simulink model "gm_Custom_DA_FIR3"  (R2023b)
settings: Solver=FixedStepDiscrete  StartTime=0.0  StopTime=10.0  RelTol=1e-3
libraries: hdlsllib x40
settings Model: Creator=adity_6z2h70p  LastModifiedBy=adity_6z2h70p
settings OptimizationCC: BlockReduction=off  ConditionallyExecuteInputs=off  DefaultParameterBehavior=Inlined  InheritOutputTypeSmallerThanSingle=on
settings DebuggingCC: AlgebraicLoopMsg=error  InheritedTsInSrcMsg=none  SingleTaskRateTransMsg=error
settings HardwareCC: ProdBitPerPointer=32  ProdBitPerSizeT=32  ProdBitPerPtrDiffT=32  ProdLargestAtomicFloat=None  ProdIntDivRoundTo=Undefined  ProdEndianess=Unspecified  ProdWordSize=32  ProdHWDeviceType=ASIC/FPGA->ASIC/FPGA  TargetBitPerPointer=64  TargetBitPerSizeT=64  TargetBitPerPtrDiffT=64  TargetLongLongMode=on  TargetIntDivRoundTo=Zero  TargetEndianess=LittleEndian  TargetWordSize=64  TargetHWDeviceType=Custom Processor->MATLAB Host Computer  ProdEqTarget=off

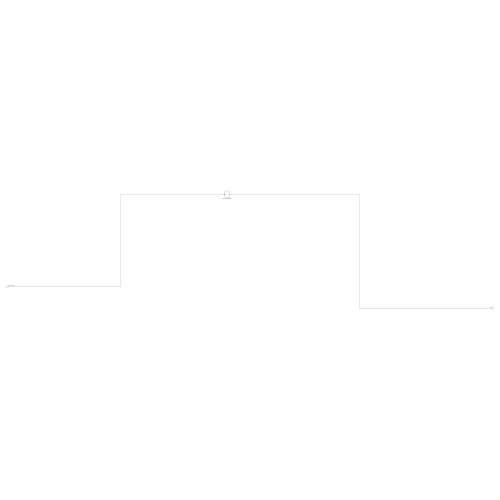
[thumbnail: Simulink's stored preview of the top-level diagram]
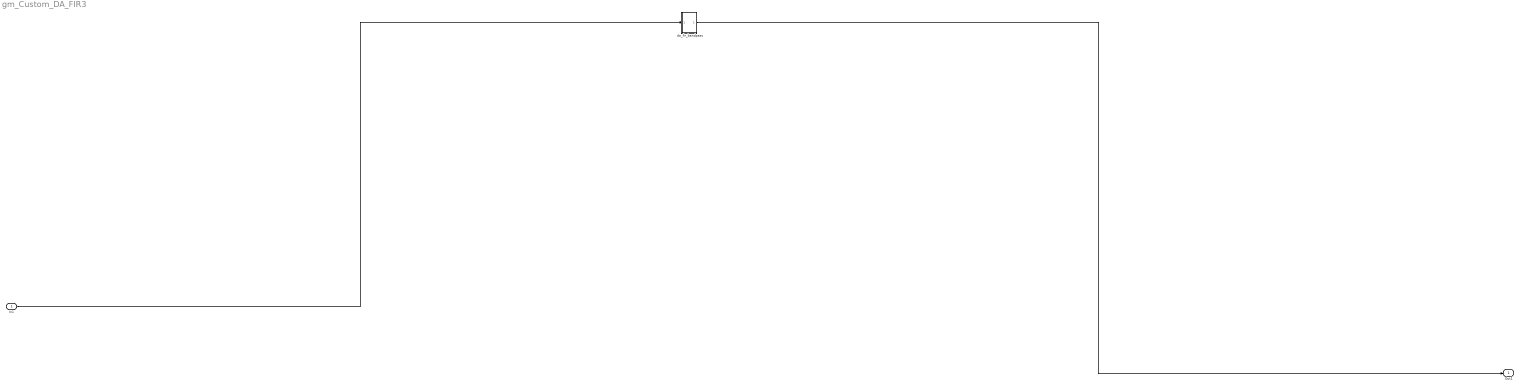
== system gm_Custom_DA_FIR3 ==
  In1 : Inport  OutDataTypeStr=fixdt(1,16,15)
  da_fir_bandpass : Subsystem
  Out1 : Outport
  wires:
  da_fir_bandpass/1(Out1) -> Out1/1
  In1/1 -> da_fir_bandpass/1(In1)

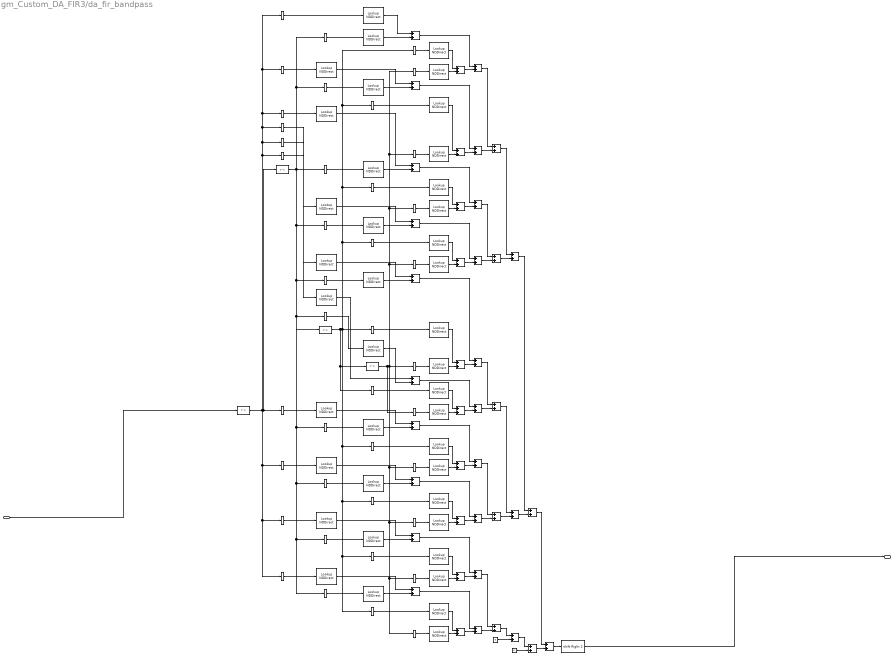
== system gm_Custom_DA_FIR3/da_fir_bandpass ==
  In1 : Inport
  Adder_S1_{1..20} (20 alike) : Sum
  Adder_S2_{1..10} (10 alike) : Sum
  Adder_S3_{1..5} (5 alike) : Sum
  Adder_S4_1 : Sum
  Adder_S4_2 : Sum
  Adder_S4_3 : Sum
  Adder_S5_1 : Sum
  Adder_S5_2 : Sum
  Adder_S6_1 : Sum
  BitSlice_Chunk_{1..40} (40 alike) : hdlsllib/Logic and Bit Operations/Bit Slice  lidx=3  ridx=0
  ConstZero_S4_3 : Constant  Value=0  OutDataTypeStr=fixdt(1,16,15)  SampleTime=-1
  ConstZero_S5_2 : Constant  Value=0  OutDataTypeStr=fixdt(1,16,15)  SampleTime=-1
  Delay_{1..4} (4 alike) : Delay  DelayLength=1
  LUT_Chunk_{1,5,8..9,11,14,18,22,26,32,35..36,39} (13 alike) : LookupNDDirect  NumberOfTableDimensions=1  Table=[0 -1 -1 -1 -1 -1 -1 -1 -1 -1 -1 -1 -1 -1 -1 -1]  TableDataTypeStr=fixdt(1,16,15)
  LUT_Chunk_10 : LookupNDDirect  NumberOfTableDimensions=1  Table=[0 0.999969482421875 0.999969482421875 0.999969482421875 0.999969482421875 0.999969482421875 0.999969482421875 0.999969482421875 -1 -1 0.999969482421875 0.999969482421875 0.999969482421875 0.999969482421875 0.999969482421875 0.999969482421875]  TableDataTypeStr=fixdt(1,16,15)
  LUT_Chunk_{3,7,12..13,16,20,24,28,34,37..38} (11 alike) : LookupNDDirect  NumberOfTableDimensions=1  Table=[0 0.999969482421875 0.999969482421875 0.999969482421875 0.999969482421875 0.999969482421875 0.999969482421875 0.999969482421875 0.999969482421875 0.999969482421875 0.999969482421875 0.999969482421875 0.999969482421875 0.999969482421875 0.999969482421875 0.999969482421875]  TableDataTypeStr=fixdt(1,16,15)
  LUT_Chunk_15 : LookupNDDirect  NumberOfTableDimensions=1  Table=[0 -1 -1 -1 -1 -1 -1 -1 0.999969482421875 -1 -1 -1 -1 -1 -1 -1]  TableDataTypeStr=fixdt(1,16,15)
  LUT_Chunk_17 : LookupNDDirect  NumberOfTableDimensions=1  Table=[0 0.999969482421875 0.999969482421875 0.999969482421875 0.999969482421875 0.999969482421875 0.999969482421875 0.999969482421875 -1 0.999969482421875 0.999969482421875 0.999969482421875 -1 0.999969482421875 0.999969482421875 0.999969482421875]  TableDataTypeStr=fixdt(1,16,15)
  LUT_Chunk_19 : LookupNDDirect  NumberOfTableDimensions=1  Table=[0 -1 -1 -1 -1 -1 -1 -1 0.999969482421875 -1 -1 -1 0.999969482421875 -1 -1 -1]  TableDataTypeStr=fixdt(1,16,15)
  LUT_Chunk_2 : LookupNDDirect  NumberOfTableDimensions=1  Table=[0 -1 0.999969482421875 -1 0.999969482421875 0.999969482421875 0.999969482421875 0.999969482421875 0.999969482421875 0.999969482421875 0.999969482421875 0.999969482421875 0.999969482421875 0.999969482421875 0.999969482421875 0.999969482421875]  TableDataTypeStr=fixdt(1,16,15)
  LUT_Chunk_21 : LookupNDDirect  NumberOfTableDimensions=1  Table=[0 0.999969482421875 0.999969482421875 0.999969482421875 -1 0.999969482421875 0.999969482421875 0.999969482421875 -1 0.999969482421875 -1 0.999969482421875 -1 0.999969482421875 -1 0.999969482421875]  TableDataTypeStr=fixdt(1,16,15)
  LUT_Chunk_23 : LookupNDDirect  NumberOfTableDimensions=1  Table=[0 -1 -1 -1 0.999969482421875 -1 -1 -1 0.999969482421875 -1 0.999969482421875 -1 0.999969482421875 0.999969482421875 0.999969482421875 -1]  TableDataTypeStr=fixdt(1,16,15)
  LUT_Chunk_25 : LookupNDDirect  NumberOfTableDimensions=1  Table=[0 0.999969482421875 0.999969482421875 0.999969482421875 -1 0.999969482421875 -1 0.999969482421875 -1 -1 -1 0.999969482421875 -1 -1 -1 -1]  TableDataTypeStr=fixdt(1,16,15)
  LUT_Chunk_27 : LookupNDDirect  NumberOfTableDimensions=1  Table=[0 -1 0.999969482421875 -1 0.999969482421875 -1 0.999969482421875 -1 0.999969482421875 0.999969482421875 0.999969482421875 0.999969482421875 0.999969482421875 0.999969482421875 0.999969482421875 0.999969482421875]  TableDataTypeStr=fixdt(1,16,15)
  LUT_Chunk_29 : LookupNDDirect  NumberOfTableDimensions=1  Table=[0 0.999969482421875 -1 0.999969482421875 -1 -1 -1 -1 -1 -1 -1 -1 -1 -1 -1 -1]  TableDataTypeStr=fixdt(1,16,15)
  LUT_Chunk_30 : LookupNDDirect  NumberOfTableDimensions=1  Table=[0 -1 -1 -1 0.999969482421875 -1 0.999969482421875 -1 0.999969482421875 -1 0.999969482421875 -1 0.999969482421875 -1 0.999969482421875 -1]  TableDataTypeStr=fixdt(1,16,15)
  LUT_Chunk_31 : LookupNDDirect  NumberOfTableDimensions=1  Table=[0 0.999969482421875 -1 -1 -1 -1 -1 -1 -1 -1 -1 -1 -1 -1 -1 -1]  TableDataTypeStr=fixdt(1,16,15)
  LUT_Chunk_33 : LookupNDDirect  NumberOfTableDimensions=1  Table=[0 -1 0.999969482421875 0.999969482421875 0.999969482421875 0.999969482421875 0.999969482421875 0.999969482421875 0.999969482421875 0.999969482421875 0.999969482421875 0.999969482421875 0.999969482421875 0.999969482421875 0.999969482421875 0.999969482421875]  TableDataTypeStr=fixdt(1,16,15)
  LUT_Chunk_4 : LookupNDDirect  NumberOfTableDimensions=1  Table=[0 0.999969482421875 -1 0.999969482421875 -1 -1 -1 -1 -1 -1 -1 -1 -1 -1 -1 -1]  TableDataTypeStr=fixdt(1,16,15)
  LUT_Chunk_40 : LookupNDDirect  NumberOfTableDimensions=1  Table=[0 -1 0 -1 0 -1 0 -1 0 -1 0 -1 0 -1 0 -1]  TableDataTypeStr=fixdt(1,16,15)
  LUT_Chunk_6 : LookupNDDirect  NumberOfTableDimensions=1  Table=[0 -1 0.999969482421875 0.999969482421875 0.999969482421875 0.999969482421875 0.999969482421875 0.999969482421875 0.999969482421875 0.999969482421875 0.999969482421875 0.999969482421875 0.999969482421875 0.999969482421875 0.999969482421875 0.999969482421875]  TableDataTypeStr=fixdt(1,16,15)
  Shift_Arithmetic_Scale : ArithShift  BitShiftNumber=2  BitShiftDirection=Right
  Out1 : Outport
  wires:
  LUT_Chunk_16/1 -> Adder_S1_8/2
  LUT_Chunk_31/1 -> Adder_S1_16/1
  Adder_S1_5/1 -> Adder_S2_3/1
  LUT_Chunk_37/1 -> Adder_S1_19/1
  BitSlice_Chunk_19/1 -> LUT_Chunk_19/1
  ConstZero_S5_2/1 -> Adder_S5_2/2
  Adder_S4_2/1 -> Adder_S5_1/2
  Adder_S2_7/1 -> Adder_S3_4/1
  LUT_Chunk_7/1 -> Adder_S1_4/1
  Adder_S1_17/1 -> Adder_S2_9/1
  Adder_S6_1/1 -> Shift_Arithmetic_Scale/1
  LUT_Chunk_8/1 -> Adder_S1_4/2
  Adder_S1_20/1 -> Adder_S2_10/2
  BitSlice_Chunk_30/1 -> LUT_Chunk_30/1
  BitSlice_Chunk_24/1 -> LUT_Chunk_24/1
  LUT_Chunk_20/1 -> Adder_S1_10/2
  LUT_Chunk_32/1 -> Adder_S1_16/2
  LUT_Chunk_21/1 -> Adder_S1_11/1
  LUT_Chunk_22/1 -> Adder_S1_11/2
  Adder_S1_10/1 -> Adder_S2_5/2
  Adder_S1_8/1 -> Adder_S2_4/2
  Adder_S1_18/1 -> Adder_S2_9/2
  Adder_S1_19/1 -> Adder_S2_10/1
  Adder_S2_10/1 -> Adder_S3_5/2
  BitSlice_Chunk_1/1 -> LUT_Chunk_1/1
  LUT_Chunk_40/1 -> Adder_S1_20/2
  LUT_Chunk_38/1 -> Adder_S1_19/2
  Adder_S3_2/1 -> Adder_S4_1/2
  LUT_Chunk_17/1 -> Adder_S1_9/1
  Adder_S1_16/1 -> Adder_S2_8/2
  LUT_Chunk_24/1 -> Adder_S1_12/2
  Adder_S3_3/1 -> Adder_S4_2/1
  Adder_S3_5/1 -> Adder_S4_3/1
  ConstZero_S4_3/1 -> Adder_S4_3/2
  LUT_Chunk_27/1 -> Adder_S1_14/1
  Adder_S2_8/1 -> Adder_S3_4/2
  LUT_Chunk_6/1 -> Adder_S1_3/2
  Adder_S5_1/1 -> Adder_S6_1/1
  Adder_S1_2/1 -> Adder_S2_1/2
  LUT_Chunk_35/1 -> Adder_S1_18/1
  LUT_Chunk_29/1 -> Adder_S1_15/1
  BitSlice_Chunk_5/1 -> LUT_Chunk_5/1
  Adder_S1_7/1 -> Adder_S2_4/1
  Adder_S1_3/1 -> Adder_S2_2/1
  LUT_Chunk_9/1 -> Adder_S1_5/1
  BitSlice_Chunk_23/1 -> LUT_Chunk_23/1
  Adder_S1_15/1 -> Adder_S2_8/1
  BitSlice_Chunk_31/1 -> LUT_Chunk_31/1
  Adder_S1_11/1 -> Adder_S2_6/1
  BitSlice_Chunk_15/1 -> LUT_Chunk_15/1
  Adder_S1_1/1 -> Adder_S2_1/1
  BitSlice_Chunk_13/1 -> LUT_Chunk_13/1
  LUT_Chunk_10/1 -> Adder_S1_5/2
  In1/1 -> Delay_1/1
  LUT_Chunk_13/1 -> Adder_S1_7/1
  BitSlice_Chunk_10/1 -> LUT_Chunk_10/1
  BitSlice_Chunk_16/1 -> LUT_Chunk_16/1
  BitSlice_Chunk_17/1 -> LUT_Chunk_17/1
  LUT_Chunk_28/1 -> Adder_S1_14/2
  BitSlice_Chunk_25/1 -> LUT_Chunk_25/1
  BitSlice_Chunk_27/1 -> LUT_Chunk_27/1
  BitSlice_Chunk_3/1 -> LUT_Chunk_3/1
  BitSlice_Chunk_18/1 -> LUT_Chunk_18/1
  LUT_Chunk_18/1 -> Adder_S1_9/2
  LUT_Chunk_33/1 -> Adder_S1_17/1
  LUT_Chunk_4/1 -> Adder_S1_2/2
  LUT_Chunk_34/1 -> Adder_S1_17/2
  BitSlice_Chunk_21/1 -> LUT_Chunk_21/1
  Adder_S1_14/1 -> Adder_S2_7/2
  BitSlice_Chunk_34/1 -> LUT_Chunk_34/1
  LUT_Chunk_36/1 -> Adder_S1_18/2
  LUT_Chunk_14/1 -> Adder_S1_7/2
  Adder_S1_4/1 -> Adder_S2_2/2
  Adder_S2_1/1 -> Adder_S3_1/1
  Adder_S1_13/1 -> Adder_S2_7/1
  Adder_S1_9/1 -> Adder_S2_5/1
  Adder_S2_9/1 -> Adder_S3_5/1
  LUT_Chunk_19/1 -> Adder_S1_10/1
  Adder_S4_1/1 -> Adder_S5_1/1
  BitSlice_Chunk_32/1 -> LUT_Chunk_32/1
  BitSlice_Chunk_4/1 -> LUT_Chunk_4/1
  BitSlice_Chunk_9/1 -> LUT_Chunk_9/1
  BitSlice_Chunk_7/1 -> LUT_Chunk_7/1
  Adder_S3_1/1 -> Adder_S4_1/1
  LUT_Chunk_23/1 -> Adder_S1_12/1
  BitSlice_Chunk_2/1 -> LUT_Chunk_2/1
  BitSlice_Chunk_28/1 -> LUT_Chunk_28/1
  BitSlice_Chunk_8/1 -> LUT_Chunk_8/1
  Adder_S2_2/1 -> Adder_S3_1/2
  LUT_Chunk_12/1 -> Adder_S1_6/2
  BitSlice_Chunk_39/1 -> LUT_Chunk_39/1
  LUT_Chunk_11/1 -> Adder_S1_6/1
  Adder_S5_2/1 -> Adder_S6_1/2
  Adder_S1_12/1 -> Adder_S2_6/2
  Adder_S1_6/1 -> Adder_S2_3/2
  BitSlice_Chunk_37/1 -> LUT_Chunk_37/1
  Adder_S2_5/1 -> Adder_S3_3/1
  Adder_S3_4/1 -> Adder_S4_2/2
  Adder_S2_6/1 -> Adder_S3_3/2
  Adder_S2_3/1 -> Adder_S3_2/1
  BitSlice_Chunk_35/1 -> LUT_Chunk_35/1
  Adder_S2_4/1 -> Adder_S3_2/2
  BitSlice_Chunk_38/1 -> LUT_Chunk_38/1
  BitSlice_Chunk_11/1 -> LUT_Chunk_11/1
  BitSlice_Chunk_20/1 -> LUT_Chunk_20/1
  BitSlice_Chunk_12/1 -> LUT_Chunk_12/1
  BitSlice_Chunk_6/1 -> LUT_Chunk_6/1
  Delay_4/1 -> BitSlice_Chunk_24/1, BitSlice_Chunk_20/1, BitSlice_Chunk_16/1, BitSlice_Chunk_12/1, BitSlice_Chunk_4/1, BitSlice_Chunk_8/1, BitSlice_Chunk_28/1, BitSlice_Chunk_32/1, BitSlice_Chunk_40/1, BitSlice_Chunk_36/1
  LUT_Chunk_5/1 -> Adder_S1_3/1
  LUT_Chunk_1/1 -> Adder_S1_1/1
  LUT_Chunk_25/1 -> Adder_S1_13/1
  BitSlice_Chunk_36/1 -> LUT_Chunk_36/1
  BitSlice_Chunk_33/1 -> LUT_Chunk_33/1
  BitSlice_Chunk_40/1 -> LUT_Chunk_40/1
  LUT_Chunk_30/1 -> Adder_S1_15/2
  Delay_2/1 -> BitSlice_Chunk_10/1, BitSlice_Chunk_6/1, BitSlice_Chunk_2/1, BitSlice_Chunk_26/1, BitSlice_Chunk_30/1, BitSlice_Chunk_34/1, BitSlice_Chunk_38/1, BitSlice_Chunk_14/1, BitSlice_Chunk_18/1, Delay_3/1, BitSlice_Chunk_22/1
  LUT_Chunk_26/1 -> Adder_S1_13/2
  BitSlice_Chunk_22/1 -> LUT_Chunk_22/1
  LUT_Chunk_39/1 -> Adder_S1_20/1
  Delay_3/1 -> BitSlice_Chunk_19/1, BitSlice_Chunk_15/1, BitSlice_Chunk_11/1, BitSlice_Chunk_3/1, BitSlice_Chunk_7/1, BitSlice_Chunk_27/1, BitSlice_Chunk_31/1, BitSlice_Chunk_39/1, BitSlice_Chunk_35/1, BitSlice_Chunk_23/1, Delay_4/1
  LUT_Chunk_3/1 -> Adder_S1_2/1
  LUT_Chunk_15/1 -> Adder_S1_8/1
  BitSlice_Chunk_26/1 -> LUT_Chunk_26/1
  BitSlice_Chunk_14/1 -> LUT_Chunk_14/1
  Adder_S4_3/1 -> Adder_S5_2/1
  BitSlice_Chunk_29/1 -> LUT_Chunk_29/1
  Shift_Arithmetic_Scale/1 -> Out1/1
  Delay_1/1 -> BitSlice_Chunk_21/1, BitSlice_Chunk_17/1, BitSlice_Chunk_13/1, BitSlice_Chunk_9/1, BitSlice_Chunk_5/1, BitSlice_Chunk_1/1, BitSlice_Chunk_25/1, Delay_2/1, BitSlice_Chunk_29/1, BitSlice_Chunk_37/1, BitSlice_Chunk_33/1
  LUT_Chunk_2/1 -> Adder_S1_1/2
